simulink model "sampleModel39"  (R2021b)
settings: Solver=VariableStepAuto  StartTime=0.0  StopTime=10.0  RelTol=1e-3
undefined symbols (not defined in the file or in its folder): Newton, Raphson
libraries: simulink x9, slpidlib x3
settings Model: Creator=user  LastModifiedBy=user

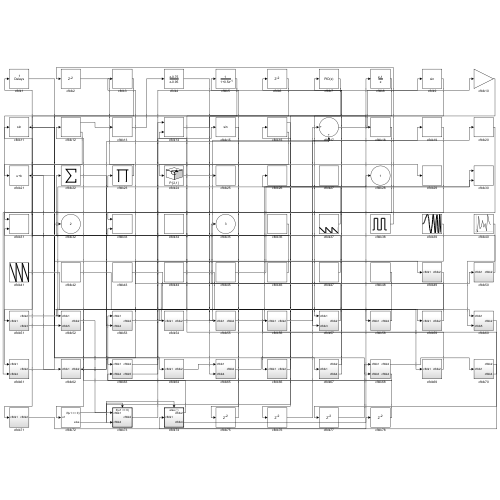
[thumbnail: Simulink's stored preview of the top-level diagram]
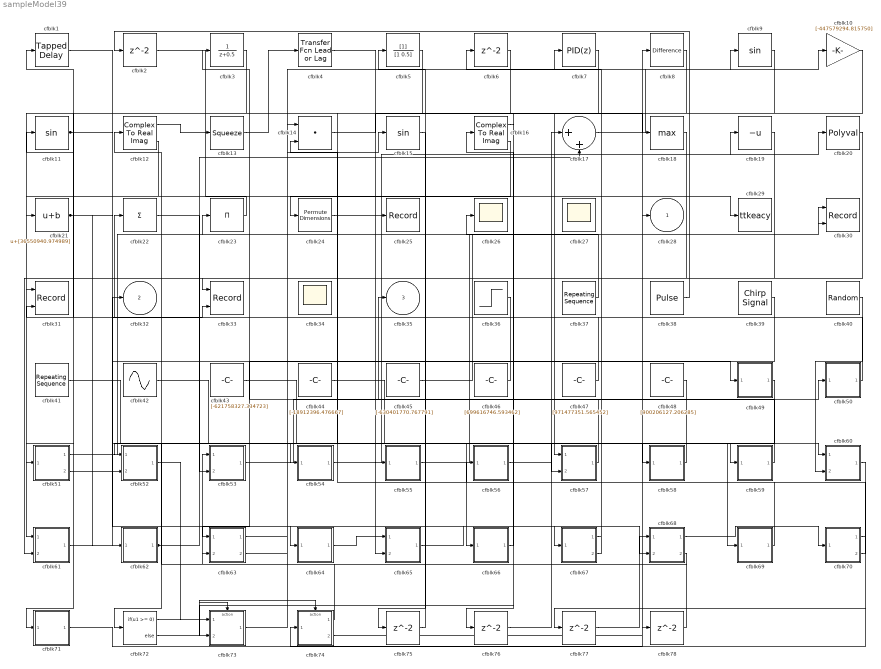
== system sampleModel39 ==
  cfblk1 : simulink/Discrete/Tapped Delay  vinit=0.0  samptime=-1  NumDelays=1  DelayOrder=Oldest  includeCurrent=off
  cfblk10 : Gain  Gain=[-447579294.815750]
  cfblk11 : Trigonometry
  cfblk12 : ComplexToRealImag
  cfblk13 : Squeeze
  cfblk14 : DotProduct  InputSameDT=on  OutDataTypeStr=Inherit: Inherit via internal rule
  cfblk15 : Trigonometry
  cfblk16 : ComplexToRealImag
  cfblk17 : Sum  Inputs=|++
  cfblk18 : MinMax  Function=max
  cfblk19 : UnaryMinus
  cfblk{2,6,75..78} (6 alike) : Delay  SampleTime=1
  cfblk20 : Polyval  Coefs=[ +2.081618890e-019, -1.441693666e-014, +4.719686976e-010, -8.536869453e-006, +1.621573104e-001, -8.087801117e+001 ]
  cfblk21 : Bias  Bias=[36550940.974989]
  cfblk22 : Sum  Inputs=+
  cfblk23 : Product  Inputs=*
  cfblk24 : PermuteDimensions
  cfblk25 : Record  FileSettingsInternal="{\"entries\":[{\"content\":{\"excelSettings\":{\"content\":{},\"type\":\"Streamout.ExcelSettings\"}},\"type\":\"Streamout.FileSettingStorage\",\"uuid\":\"b58cc6c6-0803-42f1-8792-2dce88bdd475\"}],\"packageUris\":[\"http://schema.mathworks.com/mf0/streamout_blocks/R2020a\"],\"version\":\"1.0\"}"  SignalsInternal="{\"entries\":[{\"content\":{\"signals\":[{\"content\":{\"blockPath\":[\"sampleModel39/cfblk25\"],\"channel\":[],\"dimensions\":[1,1],\"domain\":\"sampleModel39/cfblk25\",\"lineColor\":\"#64d413\",\"plots\":[1],\"port\":1,\"sid\":[\"\"],\"signalID\":1558,\"signalName\":\"cfblk24\"},\"type\":\"RecordBlkView.Signal\",\"uuid\":\"7839182a-4a85-4bd4-98e7-f1c77601c56c\"}]},\"type\":\"RecordBlkView.InputSignals\",\"uuid\":\"4cfa3398-3fab-4ab5-a008-bef041af531b\"}],\"packageUris\":[\"http://schema.mathworks.com/mf0/streamout_blocks/R2020a\"],\"version\":\"1.0\"}"  VisualizationBindings="{\"sparklinesplugin\":{\"info\":[{\"bindingParametersList\":[],\"subplotID\":1}]}}"
  cfblk26 : Scope
  cfblk27 : Scope
      settings: Floating=on
  cfblk29 : ToWorkspace  VariableName=ttkeacy  SaveFormat=Timeseries  SampleTime=-1
  cfblk3 : DiscreteTransferFcn  SampleTime=1
  cfblk30 : Record  FileSettingsInternal="{\"entries\":[{\"content\":{\"excelSettings\":{\"content\":{},\"type\":\"Streamout.ExcelSettings\"}},\"type\":\"Streamout.FileSettingStorage\",\"uuid\":\"2844526f-d2ae-473b-840a-ca48ac0b381d\"}],\"packageUris\":[\"http://schema.mathworks.com/mf0/streamout_blocks/R2020a\"],\"version\":\"1.0\"}"  Layout=[1 1]  SignalsInternal="{\"entries\":[{\"content\":{\"signals\":[{\"content\":{\"blockPath\":[\"sampleModel39/cfblk30\"],\"channel\":[],\"dimensions\":[1],\"domain\":\"sampleModel39/cfblk30\",\"lineColor\":\"#a2142f\",\"plots\":[1],\"port\":1,\"sid\":[\"\"],\"signalID\":1562,\"signalName\":\"cfblk45\"},\"type\":\"RecordBlkView.Signal\",\"uuid\":\"88290025-5d9d-4131-a71a-b32820178eb6\"},{\"content\":{\"blockPath\":[\"sampleModel39/cfblk30\"],\"channel\":[],\"dimensions\":[1],\"domain\":\"sampleModel39/cfblk30\",\"lineColor\":\"#139fff\",\"plots\":[1],\"port\":2,\"sid\":[\"\"],\"signalID\":1566,\"signalName\":\"cfblk62\"},\"type\":\"RecordBlkView.Signal\",\"uuid\":\"6245f036-5d68-4a01-a284-c2174bb31711\"}]},\"type\":\"RecordBlkView.InputSignals\",\"uuid\":\"7a530f89-876a-46fe-bee6-ac6f969f8f35\"}],\"packageUris\":[\"http://schema.mathworks.com/mf0/streamout_blocks/R2020a\"],\"version\":\"1.0\"}"  VisualizationBindings="{\"xyplotplugin\":{\"info\":[{\"series\":[{\"bindingParametersList\":[{\"parameter\":\"X-Axis\",\"signalID\":1562,\"signalName\":\"cfblk45\"},{\"parameter\":\"Y-Axis\",\"signalID\":1566,\"signalName\":\"cfblk62\"}],\"seriesID\":25258}],\"subplotID\":1}]}}"  CompatibilityTag=XY
  cfblk31 : Record  FileSettingsInternal="{\"entries\":[{\"content\":{\"excelSettings\":{\"content\":{},\"type\":\"Streamout.ExcelSettings\"}},\"type\":\"Streamout.FileSettingStorage\",\"uuid\":\"f5c27f56-3d52-4af7-b3be-966ce828023e\"}],\"packageUris\":[\"http://schema.mathworks.com/mf0/streamout_blocks/R2020a\"],\"version\":\"1.0\"}"  Layout=[1 1]  SignalsInternal="{\"entries\":[{\"content\":{\"signals\":[{\"content\":{\"blockPath\":[\"sampleModel39/cfblk31\"],\"channel\":[],\"dimensions\":[1],\"domain\":\"sampleModel39/cfblk31\",\"lineColor\":\"#a2142f\",\"plots\":[1],\"port\":1,\"sid\":[\"\"],\"signalID\":1570,\"signalName\":\"cfblk18\"},\"type\":\"RecordBlkView.Signal\",\"uuid\":\"e75b436e-d3a1-4441-a538-9306eb0c0853\"},{\"content\":{\"blockPath\":[\"sampleModel39/cfblk31\"],\"channel\":[],\"dimensions\":[1],\"domain\":\"sampleModel39/cfblk31\",\"lineColor\":\"#139fff\",\"plots\":[1],\"port\":2,\"sid\":[\"\"],\"signalID\":1574,\"signalName\":\"cfblk36\"},\"type\":\"RecordBlkView.Signal\",\"uuid\":\"d1ea4d9c-2366-4d9a-a51d-4d18cbf1c7d8\"}]},\"type\":\"RecordBlkView.InputSignals\",\"uuid\":\"481542d7-3fb9-49d9-84d3-9ee5a29a64e0\"}],\"packageUris\":[\"http://schema.mathworks.com/mf0/streamout_blocks/R2020a\"],\"version\":\"1.0\"}"  VisualizationBindings="{\"xyplotplugin\":{\"info\":[{\"series\":[{\"bindingParametersList\":[{\"parameter\":\"X-Axis\",\"signalID\":1570,\"signalName\":\"cfblk18\"},{\"parameter\":\"Y-Axis\",\"signalID\":1574,\"signalName\":\"cfblk36\"}],\"seriesID\":39622}],\"subplotID\":1}]}}"  CompatibilityTag=XY
  cfblk33 : Record  FileSettingsInternal="{\"entries\":[{\"content\":{\"excelSettings\":{\"content\":{},\"type\":\"Streamout.ExcelSettings\"}},\"type\":\"Streamout.FileSettingStorage\",\"uuid\":\"003f4ae5-0b9f-4cd6-addd-53767ee7b4eb\"}],\"packageUris\":[\"http://schema.mathworks.com/mf0/streamout_blocks/R2020a\"],\"version\":\"1.0\"}"  Layout=[1 1]  SignalsInternal="{\"entries\":[{\"content\":{\"signals\":[{\"content\":{\"blockPath\":[\"sampleModel39/cfblk33\"],\"channel\":[],\"dimensions\":[1],\"domain\":\"sampleModel39/cfblk33\",\"lineColor\":\"#a2142f\",\"plots\":[1],\"port\":1,\"sid\":[\"\"],\"signalID\":1578,\"signalName\":\"cfblk20\"},\"type\":\"RecordBlkView.Signal\",\"uuid\":\"de2a25ca-8092-4c82-aa52-e8471051a287\"},{\"content\":{\"blockPath\":[\"sampleModel39/cfblk33\"],\"channel\":[],\"dimensions\":[1],\"domain\":\"sampleModel39/cfblk33\",\"lineColor\":\"#139fff\",\"plots\":[1],\"port\":2,\"sid\":[\"\"],\"signalID\":1582,\"signalName\":\"cfblk51:2\"},\"type\":\"RecordBlkView.Signal\",\"uuid\":\"a2dc9a3d-098c-4a7c-92da-8ef66f0a6bb7\"}]},\"type\":\"RecordBlkView.InputSignals\",\"uuid\":\"72c0d555-8c1a-4978-9e71-a0ba64dd8e85\"}],\"packageUris\":[\"http://schema.mathworks.com/mf0/streamout_blocks/R2020a\"],\"version\":\"1.0\"}"  VisualizationBindings="{\"xyplotplugin\":{\"info\":[{\"series\":[{\"bindingParametersList\":[{\"parameter\":\"X-Axis\",\"signalID\":1578,\"signalName\":\"cfblk20\"},{\"parameter\":\"Y-Axis\",\"signalID\":1582,\"signalName\":\"cfblk51:2\"}],\"seriesID\":23918}],\"subplotID\":1}]}}"  CompatibilityTag=XY
  cfblk34 : Scope
      settings: Floating=on
  cfblk36 : Step  Time=[31.000000]  Before=[266568016.555120]  After=[-986625695.896016]  SampleTime=0
  cfblk37 : simulink/Sources/Repeating Sequence  rep_seq_t=[0 2]  rep_seq_y=[-570268644.650871, -837993549.178870]
  cfblk38 : DiscretePulseGenerator  PulseType=Time based  Amplitude=[-677070351.479222]  Period=[9180357.236091]  PulseWidth=5  PhaseDelay=[2.000000]
  cfblk39 : simulink/Sources/Chirp Signal  f1=[-856407649.047157]  T=[-462305338.142914]  f2=[-919866589.649345]
  cfblk4 : simulink/Discrete/Transfer Fcn Lead or Lag  PoleZ=0.95  ZeroZ=0.75  ICPrevOutput=0.0  ICPrevInput=0.0  DoSatur=off
      settings: SourceProductBaseCode=SL
  cfblk40 : UniformRandomNumber  Minimum=[-2559198968.031731]  Maximum=[9448331358.356455]  Seed=[22136054.000000]  SampleTime=0.1
  cfblk41 : simulink/Sources/Repeating Sequence  rep_seq_t=[0 2]  rep_seq_y=[201130739.618859, -127813512.701026]
  cfblk42 : Sin  Amplitude=[-652878900.698801]  Bias=[-610212034.291622]  SampleTime=0
  cfblk43 : Constant  Value=[-621758327.334723]  SampleTime=1
  cfblk44 : Constant  Value=[-18912396.476667]  SampleTime=1
  cfblk45 : Constant  Value=[-630401770.767791]  SampleTime=1
  cfblk46 : Constant  Value=[699616746.593462]  SampleTime=1
  cfblk47 : Constant  Value=[971477351.565452]  SampleTime=1
  cfblk48 : Constant  Value=[900206127.206285]  SampleTime=1
  cfblk49 : Subsystem
  cfblk5 : DiscreteFilter  SampleTime=1
  cfblk50 : Subsystem
  cfblk51 : Subsystem
  cfblk52 : Subsystem
  cfblk53 : Subsystem
  cfblk54 : Subsystem
  cfblk55 : Subsystem
  cfblk56 : Subsystem
  cfblk57 : Subsystem
  cfblk58 : Subsystem
  cfblk59 : Subsystem
  cfblk60 : Subsystem
  cfblk61 : Subsystem
  cfblk62 : Subsystem
  cfblk63 : Subsystem
  cfblk64 : Subsystem
  cfblk65 : Subsystem
  cfblk66 : Subsystem
  cfblk67 : Subsystem
  cfblk68 : Subsystem
  cfblk69 : Subsystem
  cfblk7 : slpidlib/PID Controller  Controller=PID  Form=Parallel  TimeDomain=Discrete-time  UseExternalTs=off  SampleTime=1  IntegratorMethod=Forward Euler  FilterMethod=Forward Euler  ControllerParametersSource=internal  P=1  I=1  D=0  UseFilter=on  N=100  TunerSelectOption=Transfer Function Based (PID Tuner App)  InitialConditionSource=internal  InitialConditionForIntegrator=0  InitialConditionForFilter=0  DifferentiatorICPrevScaledInput=0  ExternalReset=none  TrackingMode=off  Kt=1  LimitOutput=off  SatLimitsSource=internal  UpperSaturationLimit=inf  LowerSaturationLimit=-inf  LinearizeAsGain=off  AntiWindupMode=none  Kb=1  POutMin=[]  POutMax=[]  IOutMin=[]  IOutMax=[]  DOutMin=[]  DOutMax=[]  NOutMin=[]  NOutMax=[]  SumOutMin=[]  SumOutMax=[]  SaturationOutMin=[]  SaturationOutMax=[]  PParamMin=[]  PParamMax=[]  IParamMin=[]  IParamMax=[]  DParamMin=[]  DParamMax=[]  NParamMin=[]  NParamMax=[]  KbParamMin=[]  KbParamMax=[]  KtParamMin=[]  KtParamMax=[]  KbOutMin=[]  KbOutMax=[]  KtOutMin=[]  KtOutMax=[]  IntegratorOutMin=[]  IntegratorOutMax=[]  FilterOutMin=[]  FilterOutMax=[]  SumI1OutMin=[]  SumI1OutMax=[]  SumI2OutMin=[]  SumI2OutMax=[]  SumI3OutMin=[]  SumI3OutMax=[]  SumI4OutMin=[]  SumI4OutMax=[]  SumDOutMin=[]  SumDOutMax=[]  DifferentiatorOutMin=[]  DifferentiatorOutMax=[]  FilterDiffOutCoefMin=[]  FilterDiffOutCoefMax=[]  ReciprocalOutMin=[]  ReciprocalOutMax=[]  SumDenOutMin=[]  SumDenOutMax=[]  SumNumOutMin=[]  SumNumOutMax=[]  DivideOutMin=[]  DivideOutMax=[]  UdiffTsProdOutMin=[]  UdiffTsProdOutMax=[]  NTsProdOutMin=[]  NTsProdOutMax=[]  UintegralTsProdOutMin=[]  UintegralTsProdOutMax=[]  UngainTsProdOutMin=[]  UngainTsProdOutMax=[]  IntegratorContinuousStateAttributes=''  IntegratorStateMustResolveToSignalObject=off  IntegratorRTWStateStorageClass=Auto  FilterContinuousStateAttributes=''  FilterStateMustResolveToSignalObject=off  FilterRTWStateStorageClass=Auto  ParallelPVariant=InternalParameters  IdealPVariant=Disabled  IVariant=InternalParameters  DVariant=InternalParameters  IntegratorVariant=Discrete  SatVariant=Disabled  AWVariant=Passthrough  PCopyVariant=Disabled  TRVariant=Disabled  FdbkBlocksVariant=Forward  IdealPFdbkVariant=Disabled  SatFdbkVariant=Disabled  DerivativeFilterVariant=ForwardEulerFilter  NVariant=InternalParameters  NCopyVariant=Disabled  FilterICVariant=InternalICsFilter  IntegratorICVariant=InternalICs  ExternalResetVariant=Disabled  TRSumVariant=Passthrough  SumFdbkVariant=Disabled  SumVariant=Sum_PID  TsampFilterVariant=InternalTs  TsampNgainVariant=Passthrough  TsampIntegralVariant=Passthrough  ExternalSaturationOutDataTypeStr=Inherit: Same as second input
  cfblk70 : Subsystem
  cfblk71 : Subsystem
  cfblk72 : If  IfExpression=u1 >= 0  SampleTime=1
  cfblk73 : Subsystem  TreatAsAtomicUnit=on
  cfblk74 : Subsystem  TreatAsAtomicUnit=on
  cfblk8 : simulink/Discrete/Difference  ICPrevInput=0.0  OutMin=[]  OutMax=[]  OutDataTypeStr=Inherit: Inherit via back propagation  OutDataType=fixdt(1, 16)  OutScaling=2^-10  DoSatur=off
  cfblk9 : Trigonometry
  cfblk28 : Outport
  cfblk32 : Outport  Port=2
  cfblk35 : Outport  Port=3
  wires:
  cfblk64/1(cfblk2) -> cfblk65/1(cfblk1)
  cfblk74/1(cfblk2) -> cfblk53/1(cfblk1)
  cfblk52/1(cfblk2) -> cfblk73/1(cfblk1)
  cfblk21/1 -> cfblk62/1(cfblk1), cfblk57/2(cfblk3)
  cfblk3/1 -> cfblk61/1(cfblk1)
  cfblk23/1 -> cfblk21/1
  cfblk74/2(cfblk4) -> cfblk8/1
  cfblk37/1 -> cfblk26/1
  cfblk39/1 -> cfblk63/1(cfblk1)
  cfblk53/1(cfblk2) -> cfblk50/1(cfblk1)
  cfblk38/1 -> cfblk2/1
  cfblk48/1 -> cfblk72/1
  cfblk68/1(cfblk2) -> cfblk70/1(cfblk1)
  cfblk44/1 -> cfblk59/1(cfblk1)
  cfblk1/1 -> cfblk64/1(cfblk1)
  cfblk7/1 -> cfblk57/1(cfblk1)
  cfblk13/1 -> cfblk4/1
  cfblk2/1 -> cfblk29/1
  cfblk43/1 -> cfblk66/1(cfblk1)
  cfblk17/1 -> cfblk10/1
  cfblk45/1 -> cfblk30/1
  cfblk46/1 -> cfblk22/1
  cfblk54/1(cfblk2) -> cfblk20/1
  cfblk60/1(cfblk2) -> cfblk74/1(cfblk1)
  cfblk51/1(cfblk2) -> cfblk23/1
  cfblk24/1 -> cfblk25/1
  cfblk62/1(cfblk2) -> cfblk30/2, cfblk17/2
  cfblk56/1(cfblk2) -> cfblk19/1
  cfblk9/1 -> cfblk65/2(cfblk4)
  cfblk16/1 -> cfblk73/2(cfblk4)
  cfblk66/1(cfblk2) -> cfblk16/1
  cfblk22/1 -> cfblk60/1(cfblk1)
  cfblk16/2 -> cfblk24/1
  cfblk73/1(cfblk2) -> cfblk15/1
  cfblk57/1(cfblk2) -> cfblk3/1
  cfblk8/1 -> cfblk51/1(cfblk1)
  cfblk59/1(cfblk2) -> cfblk35/1
  cfblk42/1 -> cfblk69/1(cfblk1)
  cfblk20/1 -> cfblk33/1
  cfblk67/1(cfblk2) -> cfblk7/1
  cfblk61/1(cfblk2) -> cfblk32/1
  cfblk41/1 -> cfblk53/2(cfblk4)
  cfblk67/2(cfblk4) -> cfblk6/1
  cfblk55/1(cfblk2) -> cfblk28/1
  cfblk50/1(cfblk2) -> cfblk11/1
  cfblk12/1 -> cfblk13/1
  cfblk58/1(cfblk2) -> cfblk52/1(cfblk1)
  cfblk65/1(cfblk2) -> cfblk67/1(cfblk1)
  cfblk14/1 -> cfblk18/1
  cfblk12/2 -> cfblk71/1(cfblk1)
  cfblk63/1(cfblk2) -> cfblk14/1
  cfblk18/1 -> cfblk31/1
  cfblk47/1 -> cfblk1/1
  cfblk6/1 -> cfblk54/1(cfblk1)
  cfblk49/1(cfblk2) -> cfblk58/1(cfblk1)
  cfblk36/1 -> cfblk31/2
  cfblk51/2(cfblk3) -> cfblk33/2
  cfblk63/2(cfblk5) -> cfblk9/1
  cfblk69/1(cfblk2) -> cfblk14/2
  cfblk4/1 -> cfblk55/1(cfblk1)
  cfblk40/1 -> cfblk60/2(cfblk5)
  cfblk68/2(cfblk4) -> cfblk63/2(cfblk4)
  cfblk19/1 -> cfblk61/2(cfblk4)
  cfblk11/1 -> cfblk68/2(cfblk3), cfblk49/1(cfblk1)
  cfblk70/2(cfblk4) -> cfblk56/1(cfblk1)
  cfblk5/1 -> cfblk52/2(cfblk5)
  cfblk72/1 -> cfblk73/Action
  cfblk72/2 -> cfblk74/Action
  cfblk15/1 -> cfblk75/1
  cfblk75/1 -> cfblk5/1
  cfblk10/1 -> cfblk76/1
  cfblk76/1 -> cfblk17/1
  cfblk70/1(cfblk2) -> cfblk77/1
  cfblk77/1 -> cfblk68/1(cfblk1)
  cfblk71/1(cfblk2) -> cfblk78/1
  cfblk78/1 -> cfblk12/1

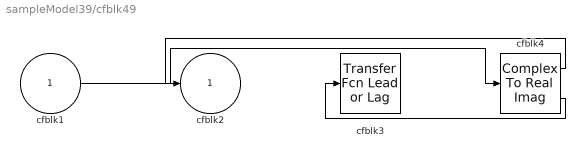
== system sampleModel39/cfblk49 ==
  cfblk1 : Inport
  cfblk3 : simulink/Discrete/Transfer Fcn Lead or Lag  PoleZ=0.95  ZeroZ=0.75  ICPrevOutput=0.0  ICPrevInput=0.0  DoSatur=off
      settings: SourceProductBaseCode=SL
  cfblk4 : ComplexToRealImag
  cfblk2 : Outport
  wires:
  cfblk1/1 -> cfblk4/1
  cfblk4/1 -> cfblk2/1
  cfblk4/2 -> cfblk3/1

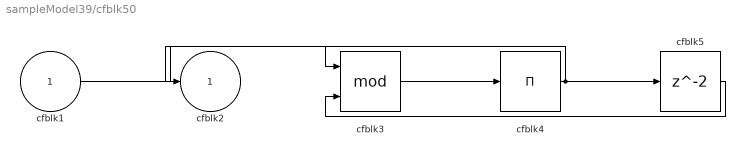
== system sampleModel39/cfblk50 ==
  cfblk1 : Inport
  cfblk3 : Math  Operator=mod  SaturateOnIntegerOverflow=on
  cfblk4 : Product  Inputs=*
  cfblk5 : Delay  SampleTime=1
  cfblk2 : Outport
  wires:
  cfblk1/1 -> cfblk3/1
  cfblk4/1 -> cfblk2/1, cfblk5/1
  cfblk3/1 -> cfblk4/1
  cfblk5/1 -> cfblk3/2

== system sampleModel39/cfblk51 ==
  cfblk1 : Inport
  cfblk2 : Outport
  cfblk3 : Outport  Port=2
  wires:
  cfblk1/1 -> cfblk2/1, cfblk3/1

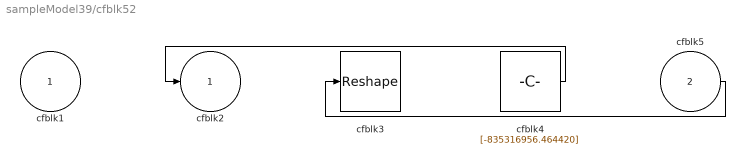
== system sampleModel39/cfblk52 ==
  cfblk1 : Inport
  cfblk5 : Inport  Port=2
  cfblk3 : Reshape
  cfblk4 : Constant  Value=[-835316956.464420]  SampleTime=1
  cfblk2 : Outport
  wires:
  cfblk4/1 -> cfblk2/1
  cfblk5/1 -> cfblk3/1

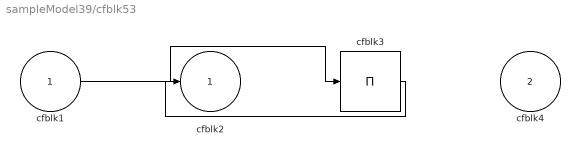
== system sampleModel39/cfblk53 ==
  cfblk1 : Inport
  cfblk4 : Inport  Port=2
  cfblk3 : Product  Inputs=*
  cfblk2 : Outport
  wires:
  cfblk1/1 -> cfblk3/1
  cfblk3/1 -> cfblk2/1

== system sampleModel39/cfblk54 ==
  cfblk1 : Inport
  cfblk3 : DiscreteZeroPole  Poles=[0 0.5]  Gain=1
  cfblk2 : Outport
  wires:
  cfblk1/1 -> cfblk3/1
  cfblk3/1 -> cfblk2/1

== system sampleModel39/cfblk55 ==
  cfblk1 : Inport
  cfblk3 : DiscreteZeroPole  Poles=[0 0.5]  Gain=1
  cfblk2 : Outport
  wires:
  cfblk1/1 -> cfblk3/1
  cfblk3/1 -> cfblk2/1

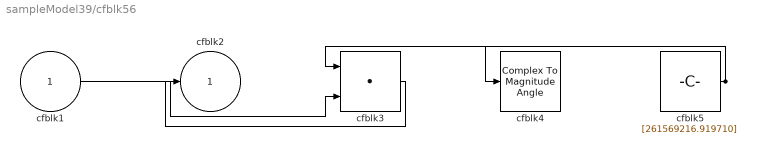
== system sampleModel39/cfblk56 ==
  cfblk1 : Inport
  cfblk3 : DotProduct  InputSameDT=on  OutDataTypeStr=Inherit: Inherit via internal rule
  cfblk4 : ComplexToMagnitudeAngle
  cfblk5 : Constant  Value=[261569216.919710]  SampleTime=1
  cfblk2 : Outport
  wires:
  cfblk5/1 -> cfblk3/1, cfblk4/1
  cfblk1/1 -> cfblk3/2
  cfblk3/1 -> cfblk2/1

== system sampleModel39/cfblk57 ==
  cfblk1 : Inport
  cfblk3 : Inport  Port=2
  cfblk2 : Outport
  wires:
  cfblk3/1 -> cfblk2/1

== system sampleModel39/cfblk58 ==
  cfblk1 : Inport
  cfblk3 : Sqrt  Operator=rSqrt  AlgorithmType=Newton-Raphson  SaturateOnIntegerOverflow=on
  cfblk4 : Constant  Value=[460223293.188000]  SampleTime=1
  cfblk2 : Outport
  wires:
  cfblk3/1 -> cfblk2/1
  cfblk4/1 -> cfblk3/1

== system sampleModel39/cfblk59 ==
  cfblk1 : Inport
  cfblk3 : simulink/Discrete/Transfer Fcn Lead or Lag  PoleZ=0.95  ZeroZ=0.75  ICPrevOutput=0.0  ICPrevInput=0.0  DoSatur=off
      settings: SourceProductBaseCode=SL
  cfblk4 : UnitDelay  HasFrameUpgradeWarning=on
  cfblk2 : Outport
  wires:
  cfblk3/1 -> cfblk4/1
  cfblk4/1 -> cfblk2/1
  cfblk1/1 -> cfblk3/1

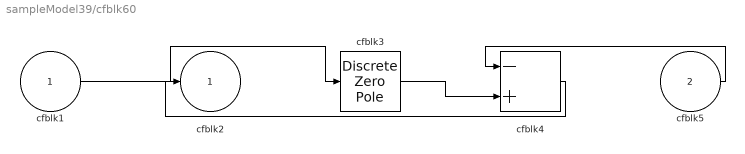
== system sampleModel39/cfblk60 ==
  cfblk1 : Inport
  cfblk5 : Inport  Port=2
  cfblk3 : DiscreteZeroPole  Poles=[0 0.5]  Gain=1
  cfblk4 : Sum  Inputs=-+
  cfblk2 : Outport
  wires:
  cfblk1/1 -> cfblk3/1
  cfblk4/1 -> cfblk2/1
  cfblk5/1 -> cfblk4/1
  cfblk3/1 -> cfblk4/2

== system sampleModel39/cfblk61 ==
  cfblk1 : Inport
  cfblk4 : Inport  Port=2
  cfblk3 : ComplexToRealImag
  cfblk2 : Outport
  wires:
  cfblk1/1 -> cfblk2/1
  cfblk4/1 -> cfblk3/1

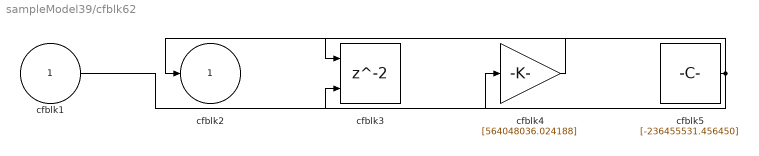
== system sampleModel39/cfblk62 ==
  cfblk1 : Inport
  cfblk3 : Delay  ShowEnablePort=on  SampleTime=1
      settings: InputPortMap=u0,e6
  cfblk4 : Gain  Gain=[564048036.024188]
  cfblk5 : Constant  Value=[-236455531.456450]  SampleTime=1
  cfblk2 : Outport
  wires:
  cfblk5/1 -> cfblk2/1, cfblk3/2
  cfblk1/1 -> cfblk4/1
  cfblk4/1 -> cfblk3/1

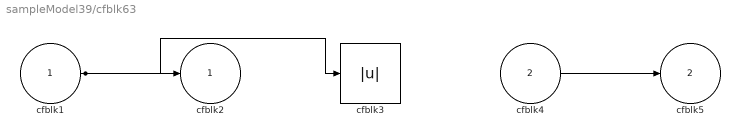
== system sampleModel39/cfblk63 ==
  cfblk1 : Inport
  cfblk4 : Inport  Port=2
  cfblk3 : Abs
  cfblk2 : Outport
  cfblk5 : Outport  Port=2
  wires:
  cfblk1/1 -> cfblk2/1, cfblk3/1
  cfblk4/1 -> cfblk5/1

== system sampleModel39/cfblk64 ==
  cfblk1 : Inport
  cfblk3 : Delay  SampleTime=1
  cfblk2 : Outport
  wires:
  cfblk1/1 -> cfblk3/1
  cfblk3/1 -> cfblk2/1

== system sampleModel39/cfblk65 ==
  cfblk1 : Inport
  cfblk4 : Inport  Port=2
  cfblk3 : PermuteDimensions
  cfblk2 : Outport
  wires:
  cfblk4/1 -> cfblk2/1
  cfblk1/1 -> cfblk3/1

== system sampleModel39/cfblk66 ==
  cfblk1 : Inport
  cfblk3 : Product  Inputs=*
  cfblk2 : Outport
  wires:
  cfblk3/1 -> cfblk2/1
  cfblk1/1 -> cfblk3/1

== system sampleModel39/cfblk67 ==
  cfblk1 : Inport
  cfblk3 : Polyval  Coefs=[ +2.081618890e-019, -1.441693666e-014, +4.719686976e-010, -8.536869453e-006, +1.621573104e-001, -8.087801117e+001 ]
  cfblk2 : Outport
  cfblk4 : Outport  Port=2
  wires:
  cfblk3/1 -> cfblk2/1, cfblk4/1
  cfblk1/1 -> cfblk3/1

== system sampleModel39/cfblk68 ==
  cfblk1 : Inport
  cfblk3 : Inport  Port=2
  cfblk2 : Outport
  cfblk4 : Outport  Port=2
  wires:
  cfblk3/1 -> cfblk4/1
  cfblk1/1 -> cfblk2/1

== system sampleModel39/cfblk69 ==
  cfblk1 : Inport
  cfblk3 : simulink/Math Operations/MinMax Running Resettable  Function=min  vinit=0.0
  cfblk2 : Outport
  wires:
  cfblk3/1 -> cfblk2/1
  cfblk1/1 -> cfblk3/1, cfblk3/2

== system sampleModel39/cfblk70 ==
  cfblk1 : Inport
  cfblk3 : DiscreteZeroPole  Poles=[0 0.5]  Gain=1
  cfblk2 : Outport
  cfblk4 : Outport  Port=2
  wires:
  cfblk1/1 -> cfblk3/1
  cfblk3/1 -> cfblk2/1, cfblk4/1

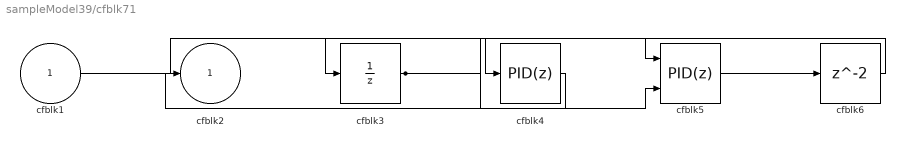
== system sampleModel39/cfblk71 ==
  cfblk1 : Inport
  cfblk3 : UnitDelay  HasFrameUpgradeWarning=on
  cfblk4 : slpidlib/PID Controller  Controller=PID  Form=Parallel  TimeDomain=Discrete-time  UseExternalTs=off  SampleTime=1  IntegratorMethod=Forward Euler  FilterMethod=Forward Euler  ControllerParametersSource=internal  P=1  I=1  D=0  UseFilter=on  N=100  TunerSelectOption=Transfer Function Based (PID Tuner App)  InitialConditionSource=internal  InitialConditionForIntegrator=0  InitialConditionForFilter=0  DifferentiatorICPrevScaledInput=0  ExternalReset=none  TrackingMode=off  Kt=1  LimitOutput=off  SatLimitsSource=internal  UpperSaturationLimit=inf  LowerSaturationLimit=-inf  LinearizeAsGain=off  AntiWindupMode=none  Kb=1  POutMin=[]  POutMax=[]  IOutMin=[]  IOutMax=[]  DOutMin=[]  DOutMax=[]  NOutMin=[]  NOutMax=[]  SumOutMin=[]  SumOutMax=[]  SaturationOutMin=[]  SaturationOutMax=[]  PParamMin=[]  PParamMax=[]  IParamMin=[]  IParamMax=[]  DParamMin=[]  DParamMax=[]  NParamMin=[]  NParamMax=[]  KbParamMin=[]  KbParamMax=[]  KtParamMin=[]  KtParamMax=[]  KbOutMin=[]  KbOutMax=[]  KtOutMin=[]  KtOutMax=[]  IntegratorOutMin=[]  IntegratorOutMax=[]  FilterOutMin=[]  FilterOutMax=[]  SumI1OutMin=[]  SumI1OutMax=[]  SumI2OutMin=[]  SumI2OutMax=[]  SumI3OutMin=[]  SumI3OutMax=[]  SumI4OutMin=[]  SumI4OutMax=[]  SumDOutMin=[]  SumDOutMax=[]  DifferentiatorOutMin=[]  DifferentiatorOutMax=[]  FilterDiffOutCoefMin=[]  FilterDiffOutCoefMax=[]  ReciprocalOutMin=[]  ReciprocalOutMax=[]  SumDenOutMin=[]  SumDenOutMax=[]  SumNumOutMin=[]  SumNumOutMax=[]  DivideOutMin=[]  DivideOutMax=[]  UdiffTsProdOutMin=[]  UdiffTsProdOutMax=[]  NTsProdOutMin=[]  NTsProdOutMax=[]  UintegralTsProdOutMin=[]  UintegralTsProdOutMax=[]  UngainTsProdOutMin=[]  UngainTsProdOutMax=[]  IntegratorContinuousStateAttributes=''  IntegratorStateMustResolveToSignalObject=off  IntegratorRTWStateStorageClass=Auto  FilterContinuousStateAttributes=''  FilterStateMustResolveToSignalObject=off  FilterRTWStateStorageClass=Auto  ParallelPVariant=InternalParameters  IdealPVariant=Disabled  IVariant=InternalParameters  DVariant=InternalParameters  IntegratorVariant=Discrete  SatVariant=Disabled  AWVariant=Passthrough  PCopyVariant=Disabled  TRVariant=Disabled  FdbkBlocksVariant=Forward  IdealPFdbkVariant=Disabled  SatFdbkVariant=Disabled  DerivativeFilterVariant=ForwardEulerFilter  NVariant=InternalParameters  NCopyVariant=Disabled  FilterICVariant=InternalICsFilter  IntegratorICVariant=InternalICs  ExternalResetVariant=Disabled  TRSumVariant=Passthrough  SumFdbkVariant=Disabled  SumVariant=Sum_PID  TsampFilterVariant=InternalTs  TsampNgainVariant=Passthrough  TsampIntegralVariant=Passthrough  ExternalSaturationOutDataTypeStr=Inherit: Same as second input
  cfblk5 : slpidlib/PID Controller (2DOF)  Controller=PID  Form=Parallel  TimeDomain=Discrete-time  UseExternalTs=off  SampleTime=1  IntegratorMethod=Forward Euler  FilterMethod=Forward Euler  ControllerParametersSource=internal  P=1  I=1  D=0  UseFilter=on  N=100  b=1  c=1  TunerSelectOption=Transfer Function Based (PID Tuner App)  InitialConditionSource=internal  InitialConditionForIntegrator=0  InitialConditionForFilter=0  DifferentiatorICPrevScaledInput=0  ExternalReset=none  TrackingMode=off  Kt=1  LimitOutput=off  SatLimitsSource=internal  UpperSaturationLimit=inf  LowerSaturationLimit=-inf  LinearizeAsGain=off  AntiWindupMode=none  Kb=1  POutMin=[]  POutMax=[]  IOutMin=[]  IOutMax=[]  DOutMin=[]  DOutMax=[]  NOutMin=[]  NOutMax=[]  bOutMin=[]  bOutMax=[]  cOutMin=[]  cOutMax=[]  SumOutMin=[]  SumOutMax=[]  SaturationOutMin=[]  SaturationOutMax=[]  PParamMin=[]  PParamMax=[]  IParamMin=[]  IParamMax=[]  DParamMin=[]  DParamMax=[]  NParamMin=[]  NParamMax=[]  bParamMin=[]  bParamMax=[]  cParamMin=[]  cParamMax=[]  KbParamMin=[]  KbParamMax=[]  KtParamMin=[]  KtParamMax=[]  KbOutMin=[]  KbOutMax=[]  KtOutMin=[]  KtOutMax=[]  IntegratorOutMin=[]  IntegratorOutMax=[]  FilterOutMin=[]  FilterOutMax=[]  SumI1OutMin=[]  SumI1OutMax=[]  SumI2OutMin=[]  SumI2OutMax=[]  SumI3OutMin=[]  SumI3OutMax=[]  SumI4OutMin=[]  SumI4OutMax=[]  SumDOutMin=[]  SumDOutMax=[]  Sum1OutMin=[]  Sum1OutMax=[]  Sum2OutMin=[]  Sum2OutMax=[]  Sum3OutMin=[]  Sum3OutMax=[]  DifferentiatorOutMin=[]  DifferentiatorOutMax=[]  FilterDiffOutCoefMin=[]  FilterDiffOutCoefMax=[]  ReciprocalOutMin=[]  ReciprocalOutMax=[]  SumDenOutMin=[]  SumDenOutMax=[]  SumNumOutMin=[]  SumNumOutMax=[]  DivideOutMin=[]  DivideOutMax=[]  UdiffTsProdOutMin=[]  UdiffTsProdOutMax=[]  NTsProdOutMin=[]  NTsProdOutMax=[]  UintegralTsProdOutMin=[]  UintegralTsProdOutMax=[]  UngainTsProdOutMin=[]  UngainTsProdOutMax=[]  IntegratorContinuousStateAttributes=''  IntegratorStateMustResolveToSignalObject=off  IntegratorRTWStateStorageClass=Auto  FilterContinuousStateAttributes=''  FilterStateMustResolveToSignalObject=off  FilterRTWStateStorageClass=Auto  ParallelPVariant=InternalParameters  IdealPVariant=Disabled  IVariant=InternalParameters  DVariant=InternalParameters  bVariant=InternalParameters  cVariant=InternalParameters  IntegratorVariant=Discrete  SatVariant=Disabled  AWVariant=Passthrough  PCopyVariant=Disabled  TRVariant=Disabled  FdbkBlocksVariant=Forward  IdealPFdbkVariant=Disabled  SatFdbkVariant=Disabled  DerivativeFilterVariant=ForwardEulerFilter  NVariant=InternalParameters  NCopyVariant=Disabled  FilterICVariant=InternalICsFilter  IntegratorICVariant=InternalICs  ExternalResetVariant=Disabled  TRSumVariant=Passthrough  SumFdbkVariant=Disabled  SumVariant=Sum_PID  TsampFilterVariant=InternalTs  TsampNgainVariant=Passthrough  TsampIntegralVariant=Passthrough  ExternalSaturationOutDataTypeStr=Inherit: Same as second input
      settings: SourceProductBaseCode=SL
  cfblk6 : Delay  SampleTime=1
  cfblk2 : Outport
  wires:
  cfblk1/1 -> cfblk4/1
  cfblk4/1 -> cfblk2/1
  cfblk3/1 -> cfblk5/1, cfblk5/2
  cfblk5/1 -> cfblk6/1
  cfblk6/1 -> cfblk3/1

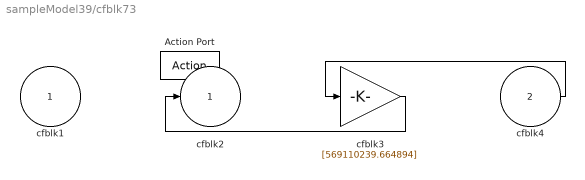
== system sampleModel39/cfblk73 ==
  cfblk1 : Inport
  cfblk4 : Inport  Port=2
  Action Port : ActionPort  ActionPortLabel=if(u1 >= 0)
  cfblk3 : Gain  Gain=[569110239.664894]
  cfblk2 : Outport
  wires:
  cfblk3/1 -> cfblk2/1
  cfblk4/1 -> cfblk3/1

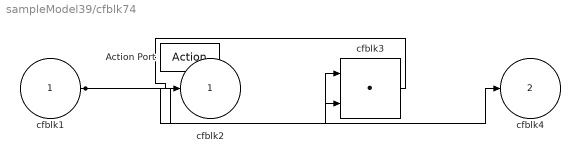
== system sampleModel39/cfblk74 ==
  cfblk1 : Inport
  Action Port : ActionPort  ActionPortLabel=else
  cfblk3 : DotProduct  InputSameDT=on  OutDataTypeStr=Inherit: Inherit via internal rule
  cfblk2 : Outport
  cfblk4 : Outport  Port=2
  wires:
  cfblk1/1 -> cfblk4/1, cfblk3/1, cfblk3/2
  cfblk3/1 -> cfblk2/1
